simulink model "qqqq"  (R2017b)
settings: Solver=VariableStepAuto  StartTime=0.0  StopTime=10.0  RelTol=1e-3
values from neighbouring files (symbols this model uses):
  d = y(end)    [main.m]
settings Model: Creator=Chiger  LastModifiedBy=Chiger

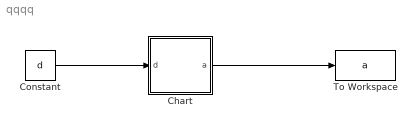
== system qqqq ==
  Chart : Stateflow chart  TreatAsAtomicUnit=on
  Constant : Constant  Value=d
  To Workspace : ToWorkspace  VariableName=a  SaveFormat=Timeseries  SampleTime=-1
  wires:
  Constant/1 -> Chart/1(d)
  Chart/1(a) -> To Workspace/1

== stateflow chart qqqq/Chart ==
  state L
    entry: a=1;
  state R
    entry: a=2;
  state N
  (default) -> (junction 3) [order 1]
  L -> (junction 9) : {a=1}
  (junction 3) -> L [order 1] : [d>10]
  (junction 3) -> R [order 2] : [d<-10]
  (default) -> N [order 2]
  N -> (junction 9) : {a=3}
  R -> (junction 9) : {a=2}
  data: d input double; a output double
